simulink model "model_metoda_svf"  (R2023b)
settings: Solver=VariableStepAuto  StartTime=0.0  StopTime=t(end)  RelTol=1e-3
InitFcn:
  | load("dane_weryfikacyjne.mat")
  | load("parametry_SVF.mat")
  | 
  | u_ts = [t u];
  | % u_ts = timeseries(u,t);
  | % u_ts = setinterpmethod(u_ts, 'zoh');
  | 
  | y_ts = [t y];
values from neighbouring files (symbols this model uses):
  parametry_SVF = pinv(Phi)*yppF    [s_05_indentyfikacja_fitrSVF.m]
  Tp = 0.01    [s_01_podzial_danych.m]    (also in s_02_analiza_czestotliwosciowa.m)
  y = RWP(:,2)    [animacja_danych.m]    (also in s_01_podzial_danych.m = y_full((N - N_cut+1):end); s_02_analiza_czestotliwosciowa.m; transmorata_wejscia.m)
settings Model: Creator=Tymo  LastModifiedBy=Tymo

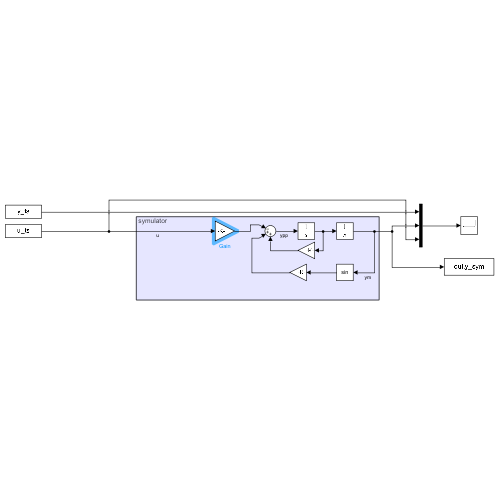
[thumbnail: Simulink's stored preview of the top-level diagram]
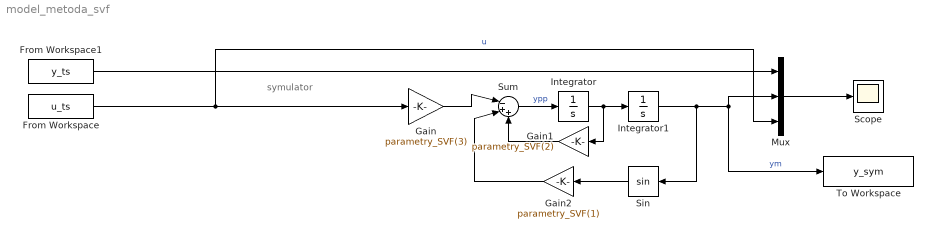
== system model_metoda_svf ==
  note: symulator
  From Workspace : FromWorkspace  VariableName=u_ts  SampleTime=Tp
  From Workspace1 : FromWorkspace  VariableName=y_ts  SampleTime=Tp
  Gain : Gain  Gain=parametry_SVF(3)
  Gain1 : Gain  Gain=parametry_SVF(2)
  Gain2 : Gain  Gain=parametry_SVF(1)
  Integrator : Integrator
  Integrator1 : Integrator
  Mux : Mux  Inputs=3
  Scope : Scope
  Sin : Trigonometry
  Sum : Sum  Inputs=|-++
  To Workspace : ToWorkspace  VariableName=y_sym  SaveFormat=Timeseries  SampleTime=-1
  wires:
  Gain/1 -> Sum/1
  Gain2/1 -> Sum/2
  Sum/1 -> Integrator/1  "ypp"
  Integrator/1 -> Gain1/1, Integrator1/1
  Integrator1/1 -> Sin/1, To Workspace/1, Mux/2  "ym"
  Mux/1 -> Scope/1
  From Workspace1/1 -> Mux/1
  From Workspace/1 -> Mux/3, Gain/1  "u"
  Sin/1 -> Gain2/1
  Gain1/1 -> Sum/3
